simulink model "qpsk_receiver_sample"  (R2019a)
settings: Solver=VariableStepAuto  StartTime=0.0  StopTime=1/0  RelTol=1e-3
undefined symbols (not defined in the file): sdrqpskrx, startfcn_spectrum_analyzer
libraries: commrfcorlib x2, commsync2 x2, dspstat3 x1, commrflib2 x1, sdrrlib x1, commfilt2 x1
settings Model: Creator=irfan.ullah  LastModifiedBy=irfan.ullah

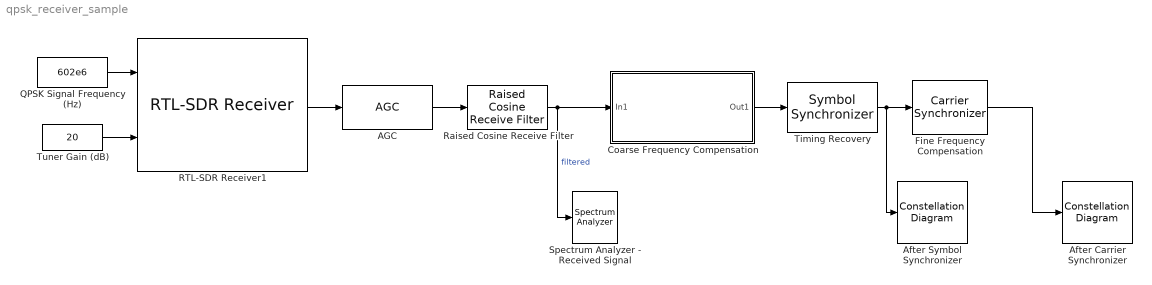
== system qpsk_receiver_sample ==
  AGC : commrfcorlib/AGC  LegacyMode=off  DetectorMethod=Rectifier  LoopMethod=Linear  UpdatePeriod=100  StepSize=0.1  AdaptationStepSize=0.01  DesiredOutputPower=sdrqpskrx.DesiredPower  AveragingLength=sdrqpskrx.AveragingLength  MaximumGain=30  MaxPowerGain=sdrqpskrx.MaxPowerGain  GainOutputPort=off  InputPowerOutputPort=off  SimulateUsing=Code generation
      settings: SourceProductName=Communications Toolbox
  After Carrier Synchronizer : ConstellationDiagram  Tag=ScatterPlot
  After Symbol Synchronizer : ConstellationDiagram  Tag=ScatterPlot
  Coarse Frequency Compensation : Subsystem
      mask Display: fprintf('Coarse Frequency\nCompensation')
  Fine Frequency Compensation : commsync2/Carrier Synchronizer  Modulation=QPSK  ModulationPhaseOffset=Auto  CustomPhaseOffset=0  SamplesPerSymbol=sdrqpskrx.Interpolation/sdrqpskrx.Decimation  DampingFactor=1  NormalizedLoopBandwidth=0.01  EstimatedPhaseErrorOutputPort=off  SimulateUsing=Code generation
      settings: SourceProductName=Communications Toolbox
  "QPSK Signal Frequency (Hz) " : Constant  Value=602e6
  RTL-SDR Receiver1 : sdrrlib/RTL-SDR Receiver  IPAddress=0  CenterFrequencySource=Input port  CenterFrequency=433.9e6  GainSource=Input port  Gain=15  ADCRate=240e3  FrequencyCorrection=0  LostSamplesOutputPort=off  LatencyOutputPort=off  OutputDataType=single  FrameLength=4096  EnableBurstMode=off  NumFramesInBurst=20  sobjType=sdrr.internal.SDRRTLReceiverSL  dataUDPPort=-1  ctrlUDPPort=-1  subDeviceList=nosubdev  sdrBlockType=SDRBlockTypeSLT.SDRRxBlock  requester=UNUSED_BY_SFCN  sdrExecutionMode=SDRExecutionModeSLT.ExecModeHW  BypassUserLogic=off  DecimatorSelect=DDC decimator  SourceSelect=RF data  SineAmplitude=16000  EnableInternalClock=off  BypassIQBalance=off  IFBandwidth=40e6  ADCRateSource=Dialog  IntermediateFrequency=0  DecimationFactorSource=Dialog  DecimationFactor=512  RFFrequencyIsTunable=logical(1)  SampleTime=(4096)/(240e3)  IFBandwidthSource=Dialog  SineFrequency=30000  BypassDCBlockingFilter=off  IntermediateFrequencySource=Dialog  IQBalanceCoefficients=64  SkipAllHardwareResetAndInitialization=off  EnableIQCalibrationTable=on  CacheIQCalibrationTable=off  EnableOffsetTuning=off  EnableRTLAGC=off  EnableTestMode=off  EnableTunerAGC=off  FrequencyCorrectionSource=Dialog  NumMLBuffers=128  NumUSBBuffers=16  RTLCrystalFrequency=28800000  TunerCrystalFrequency=28800000
      settings: SourceProductName=Communications Toolbox Support Package for RTL-SDR Radio  SourceProductBaseCode=RTLSDR
  Raised Cosine Receive Filter : commfilt2/Raised Cosine Receive Filter  filtType=Square root  R=sdrqpskrx.RolloffFactor  filtSpan=sdrqpskrx.RaisedCosineFilterSpan  N=sdrqpskrx.Interpolation  downFactor=sdrqpskrx.Decimation  downOffset=0  filterGain=1  InputProcessing=Columns as channels (frame based)  RateOptions=Enforce single-rate processing  framing=Mute  checkCoeff=off  variableName=rcRxFilt  currentFiltSpan=10  D=5  inputOffset=0  sampMode=Mute  saveAsFlag=0  rateMode=Downsampling  checkGain=Normalized  launchFVT=on  roundingMode=Floor  overflowMode=off  coeffDataTypeStr=Inherit: Same word length as input  coeffMin=[]  coeffMax=[]  coeffLastDataTypeStr=Inherit: Same word length as input  accumDataTypeStr=Inherit: Same as product output  accumLastDataTypeStr=Inherit: Same as product output  outputDataTypeStr=Inherit: Same as accumulator  outputMin=[]  outputMax=[]  outputLastDataTypeStr=Inherit: Same as accumulator
      settings: SourceProductName=Communications Toolbox
  Spectrum Analyzer - Received Signal : SpectrumAnalyzer  StartFcn=startfcn_spectrum_analyzer;
  Timing Recovery : commsync2/Symbol Synchronizer  Modulation=PAM/PSK/QAM  TimingErrorDetector=Gardner (non-data-aided)  SamplesPerSymbol=sdrqpskrx.Interpolation/sdrqpskrx.Decimation  DampingFactor=1  NormalizedLoopBandwidth=0.01  DetectorGain=sdrqpskrx.TimingErrorDetectorGain  TimingErrorOutputPort=off  SimulateUsing=Code generation
      settings: SourceProductName=Communications Toolbox  SourceProductBaseCode=CM
  Tuner Gain (dB) : Constant  Value=20
  wires:
  "QPSK Signal Frequency (Hz) "/1 -> RTL-SDR Receiver1/1
  Tuner Gain (dB)/1 -> RTL-SDR Receiver1/2
  RTL-SDR Receiver1/1 -> AGC/1
  AGC/1 -> Raised Cosine Receive Filter/1
  Raised Cosine Receive Filter/1 -> Coarse Frequency Compensation/1(In1), Spectrum Analyzer - Received Signal/1  "filtered"
  Coarse Frequency Compensation/1(Out1) -> Timing Recovery/1
  Timing Recovery/1 -> After Symbol Synchronizer/1, Fine Frequency Compensation/1
  Fine Frequency Compensation/1 -> After Carrier Synchronizer/1

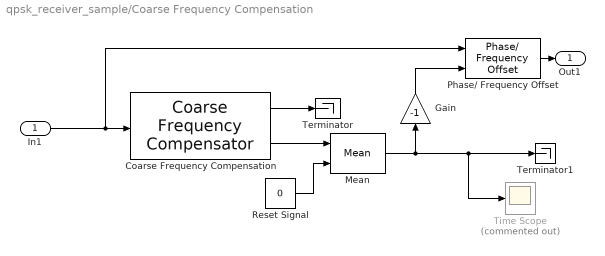
== system qpsk_receiver_sample/Coarse Frequency Compensation ==
  In1 : Inport
  Coarse Frequency Compensation : commrfcorlib/Coarse Frequency Compensator  Modulation=QPSK  Algorithm=Correlation-based  FrequencyResolution=25  MaximumFrequencyOffset=12.5e3  SamplesPerSymbol=4  EstimatedFreqOffsetPort=on  SimulateUsing=Code generation
      settings: SourceProductName=Communications Toolbox  SourceProductBaseCode=CM
  Gain : Gain  Gain=-1
  Mean : dspstat3/Mean  run=on  InputProcessing=Columns as channels (frame based)  reset_popup=Either edge  directionMode=Each column  dimension=1  roiEnable=off  roiType=Rectangles  roiPortion=Entire ROI  roiOutput=Individual statistics for each ROI  roiFlag=off  roundingMode=Floor  overflowMode=off  outputDataTypeStr=Inherit: Same as accumulator  outputMin=[]  outputMax=[]  outputLastDataTypeStr=Inherit: Same as accumulator
  Phase/ Frequency Offset : commrflib2/Phase// Frequency Offset  phaseOffset=0  freqPort=on  freqOffset=0
      settings: SourceProductName=Communications Toolbox
  Reset Signal : Constant  Value=0
  Terminator : Terminator
  Terminator1 : Terminator
  Time Scope : Scope  Commented=on
  Out1 : Outport
  wires:
  In1/1 -> Phase/ Frequency Offset/1, Coarse Frequency Compensation/1
  Phase/ Frequency Offset/1 -> Out1/1
  Mean/1 -> Time Scope/1, Terminator1/1, Gain/1
  Coarse Frequency Compensation/2 -> Mean/1
  Coarse Frequency Compensation/1 -> Terminator/1
  Gain/1 -> Phase/ Frequency Offset/2
  Reset Signal/1 -> Mean/2
